simulink model "PP_simulink_Sily"  (R2024b)
settings: Solver=ode1  StartTime=0.0  StopTime=1  FixedStep=0.005  RelTol=1e-3
values from neighbouring files (symbols this model uses):
  init_int_dref = -Ki\((Uinit-Us)+Kp*(Xinit_ss-Xs))    [PP_matlab_client_Sily.m]
  Ki = K_ex_other_angles(:, 17:20)    [PP_koeficienty.m]
  Kp = K_ex_other_angles(:, 1:16)    [PP_koeficienty.m]
  L_obs = place(Ac', Cc', poles_obs)'    [PP_koeficienty.m]
undefined symbols (not defined in the file or in its folder): b_moment, d, g, Ip, Ixx, Iyy, Izz, k_thrust, l, M, m, Us, Xinit_ss, Xs
libraries: simulink_extras x6
settings Model: Creator=yaozhong.zhang  LastModifiedBy=Admin
settings DebuggingCC: UnconnectedInputMsg=warning  UnconnectedOutputMsg=warning  UnconnectedLineMsg=warning
settings ModelReferenceCC: EnableRefExpFcnMdlSchedulingChecks=on
settings RTWCC: GPUComputeCapability=3.5

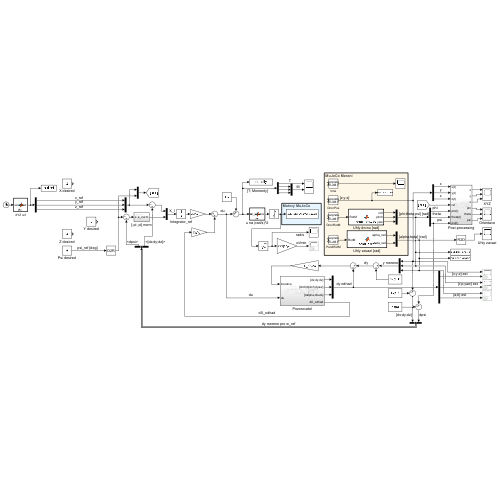
[thumbnail: Simulink's stored preview of the top-level diagram]
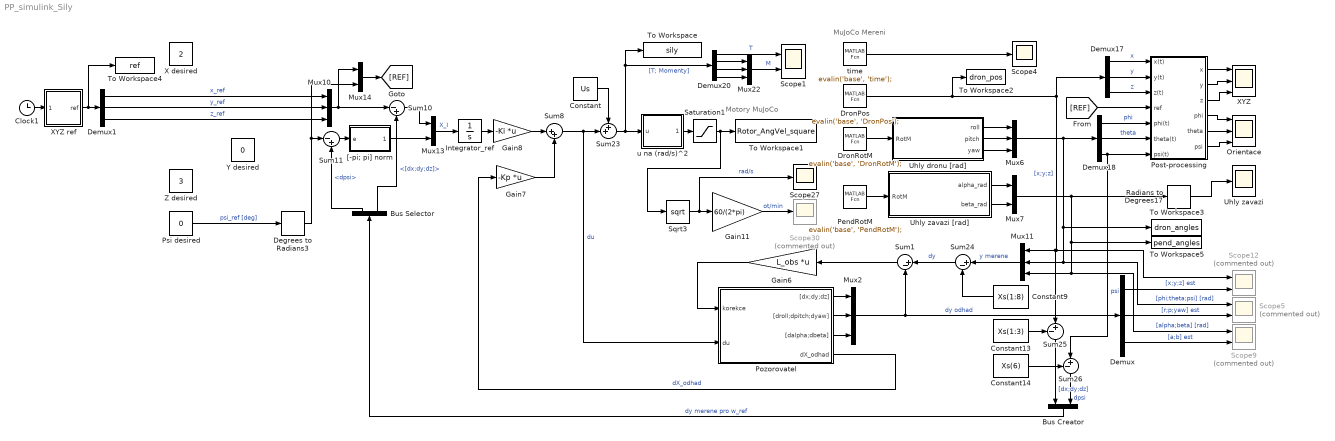
== system PP_simulink_Sily ==
  note: Motory MuJoCo
  note: MuJoCo Mereni
  Bus Creator : BusCreator  Inputs=2
  Bus Selector : BusSelector  OutputSignals=dpsi,[dx;dy;dz]
  Clock1 : Clock
  Constant : Constant  Value=Us
  Constant13 : Constant  Value=Xs(1:3)
  Constant14 : Constant  Value=Xs(6)
  Constant9 : Constant  Value=Xs(1:8)
  Degrees to Radians3 : simulink_extras/Transformations/Degrees to Radians
  Demux{,1,17..18} (4 alike) : Demux  Outputs=3
  Demux20 : Demux
  DronPos : MATLABFcn  MATLABFcn=evalin('base', 'DronPos');  OutputDimensions=[3,1]  Output1D=off
  DronRotM : MATLABFcn  MATLABFcn=evalin('base', 'DronRotM');  OutputDimensions=[3,3]  Output1D=off
  Gain11 : Gain  Gain=60/(2*pi)
  Gain6 : Gain  Gain=L_obs  Multiplication=Matrix(K*u)
  Gain7 : Gain  Gain=-Kp  Multiplication=Matrix(K*u)
  Gain8 : Gain  Gain=-Ki  Multiplication=Matrix(K*u)
  Integrator_ref : Integrator  InitialCondition=init_int_dref
  Mux{2,6,10..11,22} (5 alike) : Mux  Inputs=3
  Mux13 : Mux  Inputs=2
  Mux14 : Mux  Inputs=2
  Mux7 : Mux  Inputs=2
  Orientace : Scope  NumInputPorts=3
  PendRotM : MATLABFcn  MATLABFcn=evalin('base', 'PendRotM');  OutputDimensions=[3,3]  Output1D=off
  Post-processing : Subsystem
  Pozorovatel : Subsystem
  Psi desired : Constant  Value=0
  Radians to Degrees17 : simulink_extras/Transformations/Radians to Degrees
  Saturation1 : Saturate  UpperLimit=1976^2  LowerLimit=0
  Scope1 : Scope  NumInputPorts=2
  Scope12 : Scope  Commented=on  NumInputPorts=2
  Scope27 : Scope
  Scope30 : Scope  Commented=on
  Scope4 : Scope
  Scope5 : Scope  Commented=on  NumInputPorts=2
  Scope9 : Scope  Commented=on  NumInputPorts=2
  Sqrt3 : Sqrt
  Sum1 : Sum  Inputs=|+-
  Sum10 : Sum  Inputs=|-+
  Sum11 : Sum  Inputs=|-+
  Sum23 : Sum  Inputs=++|
  Sum24 : Sum  Inputs=|+-
  Sum25 : Sum  Inputs=-+|
  Sum26 : Sum  Inputs=-+|
  Sum8 : Sum  Inputs=|++
  To Workspace : ToWorkspace  VariableName=sily  SaveFormat=Timeseries  SampleTime=-1
  To Workspace1 : ToWorkspace  VariableName=Rotor_AngVel_square  SampleTime=-1
  To Workspace2 : ToWorkspace  VariableName=dron_pos  SaveFormat=Timeseries  SampleTime=-1
  To Workspace3 : ToWorkspace  VariableName=dron_angles  SaveFormat=Timeseries  SampleTime=-1
  To Workspace4 : ToWorkspace  VariableName=ref  SaveFormat=Timeseries  SampleTime=-1
  To Workspace5 : ToWorkspace  VariableName=pend_angles  SaveFormat=Timeseries  SampleTime=-1
  Uhly dronu [rad] : MATLAB Function  TreatAsAtomicUnit=on
  Uhly zavazi : Scope
  Uhly zavazi [rad] : MATLAB Function  TreatAsAtomicUnit=on
  X desired : Constant  Value=2
  XYZ : Scope  NumInputPorts=3
  XYZ ref : MATLAB Function  TreatAsAtomicUnit=on
  Y desired : Constant  Value=0
  Z desired : Constant  Value=3
  "[-pi; pi] norm" : Subsystem
  time : MATLABFcn  MATLABFcn=evalin('base', 'time');  Output1D=off
  u na (rad/s)^2 : MATLAB Function  TreatAsAtomicUnit=on
  wires:
  Demux/1 -> Scope12/2  "[x;y;z] est"
  Demux/2 -> Scope5/2  "[r;p;yaw] est"
  Demux/3 -> Scope9/2  "[a;b] est"
  Mux6/1 -> Mux11/2, Scope5/1, To Workspace3/1, Demux18/1  "[phi;theta;psi] [rad]"
  Gain7/1 -> Sum8/2
  Post-processing/1(x) -> XYZ/1
  Integrator_ref/1 -> Gain8/1
  Post-processing/5(theta) -> Orientace/2
  Degrees to Radians3/1 -> Mux14/2, Sum11/1
  Post-processing/4(phi) -> Orientace/1
  [REF] -> Post-processing/4(ref)
  Mux13/1 -> Integrator_ref/1  "X_I"
  Demux17/1 -> Post-processing/1(x(t))  "x"
  Radians to Degrees17/1 -> Uhly zavazi/1
  Mux22/1 -> Scope1/2  "M"
  Gain11/1 -> Scope30/1  "ot/min"
  Post-processing/6(psi) -> Orientace/3
  Demux18/1 -> Post-processing/5(phi(t))  "phi"
  Sqrt3/1 -> Scope27/1, Gain11/1  "rad/s"
  Pozorovatel/4(dX_odhad) -> Gain7/1  "dX_odhad"
  Demux18/3 -> Post-processing/7(psi(t)), Sum26/2  "psi"
  Demux1/3 -> Mux10/3  "z_ref"
  Post-processing/3(z) -> XYZ/3
  "[-pi; pi] norm"/1(e_norm) -> Mux13/2
  Sum10/1 -> Mux13/1
  Demux18/2 -> Post-processing/6(theta(t))  "theta"
  Psi desired/1 -> Degrees to Radians3/1  "psi_ref [deg]"
  Demux20/4 -> Mux22/3
  Demux20/1 -> Scope1/1  "T"
  Post-processing/2(y) -> XYZ/2
  Sum23/1 -> To Workspace/1, Demux20/1, u na (rad/s)^2/1(u)  "[T; Momenty]"
  Bus Creator/1 -> Bus Selector/1  "dy merene pro w_ref"
  Gain8/1 -> Sum8/1
  Demux1/1 -> Mux10/1  "x_ref"
  Sum11/1 -> "[-pi; pi] norm"/1(e)
  Demux20/3 -> Mux22/2
  Demux17/3 -> Post-processing/3(z(t))  "z"
  Mux10/1 -> Mux14/1, Sum10/1
  DronPos/1 -> To Workspace2/1, Demux17/1, Mux11/1, Sum25/2, Scope12/1  "[x;y;z]"
  Demux1/2 -> Mux10/2  "y_ref"
  Demux20/2 -> Mux22/1
  Demux17/2 -> Post-processing/2(y(t))  "y"
  u na (rad/s)^2/1(wi_square) -> Saturation1/1
  Saturation1/1 -> Sqrt3/1, To Workspace1/1
  Uhly zavazi [rad]/1(alpha_rad) -> Mux7/1
  time/1 -> Scope4/1
  Uhly zavazi [rad]/2(beta_rad) -> Mux7/2
  Mux7/1 -> Radians to Degrees17/1, Mux11/3, Scope9/1, To Workspace5/1  "[alpha;beta] [rad]"
  DronRotM/1 -> Uhly dronu [rad]/1(RotM)
  Uhly dronu [rad]/1(roll) -> Mux6/1
  Uhly dronu [rad]/3(yaw) -> Mux6/3
  Uhly dronu [rad]/2(pitch) -> Mux6/2
  PendRotM/1 -> Uhly zavazi [rad]/1(RotM)
  Mux14/1 -> [REF]
  Sum25/1 -> Bus Creator/1  "[dx;dy;dz]"
  Constant13/1 -> Sum25/1
  Constant14/1 -> Sum26/1
  Sum26/1 -> Bus Creator/2  "dpsi"
  Bus Selector/1 -> Sum11/2  "<dpsi>"
  Bus Selector/2 -> Sum10/2  "<[dx;dy;dz]>"
  Constant/1 -> Sum23/1
  Sum8/1 -> Pozorovatel/2(du), Sum23/2  "du"
  Sum24/1 -> Sum1/1  "dy"
  Mux2/1 -> Sum1/2, Demux/1  "dy odhad"
  Gain6/1 -> Pozorovatel/1(korekce)
  Mux11/1 -> Sum24/1  "y merene"
  Constant9/1 -> Sum24/2
  Sum1/1 -> Gain6/1
  Pozorovatel/1("[dx;dy;dz]") -> Mux2/1
  Pozorovatel/2("[droll;dpitch;dyaw]") -> Mux2/2
  Pozorovatel/3("[dalpha;dbeta]") -> Mux2/3
  Clock1/1 -> XYZ ref/1(simtime)
  XYZ ref/1(ref) -> To Workspace4/1, Demux1/1

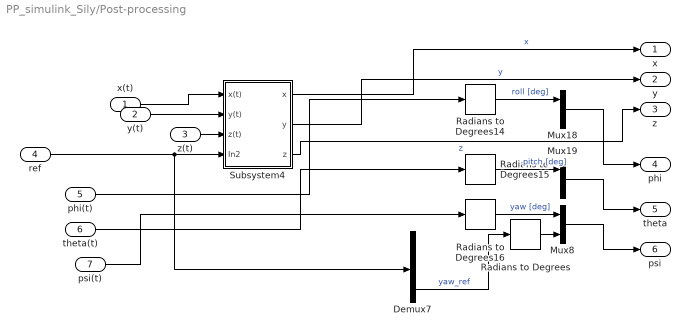
== system PP_simulink_Sily/Post-processing ==
  x(t) : Inport
  y(t) : Inport  Port=2
  z(t) : Inport  Port=3
  ref : Inport  Port=4
  phi(t) : Inport  Port=5
  theta(t) : Inport  Port=6
  psi(t) : Inport  Port=7
  Demux7 : Demux
  Mux18 : Mux  Inputs=2
  Mux19 : Mux  Inputs=2
  Mux8 : Mux  Inputs=2
  Radians to Degrees{,14..16} (4 alike) : simulink_extras/Transformations/Radians to Degrees
  Subsystem4 : Subsystem
  x : Outport
  y : Outport  Port=2
  z : Outport  Port=3
  phi : Outport  Port=4
  theta : Outport  Port=5
  psi : Outport  Port=6
  wires:
  Radians to Degrees16/1 -> Mux8/1  "yaw [deg]"
  ref/1 -> Subsystem4/4(In2), Demux7/1
  Demux7/4 -> Radians to Degrees/1  "yaw_ref"
  theta(t)/1 -> Radians to Degrees15/1
  Mux18/1 -> phi/1
  Subsystem4/3(z) -> z/1  "z"
  Radians to Degrees14/1 -> Mux18/1  "roll [deg]"
  Radians to Degrees15/1 -> Mux19/1  "pitch [deg]"
  Subsystem4/2(y) -> y/1  "y"
  x(t)/1 -> Subsystem4/1(x(t))
  y(t)/1 -> Subsystem4/2(y(t))
  psi(t)/1 -> Radians to Degrees16/1
  phi(t)/1 -> Radians to Degrees14/1
  Subsystem4/1(x) -> x/1  "x"
  Mux8/1 -> psi/1
  z(t)/1 -> Subsystem4/3(z(t))
  Mux19/1 -> theta/1
  Radians to Degrees/1 -> Mux8/2

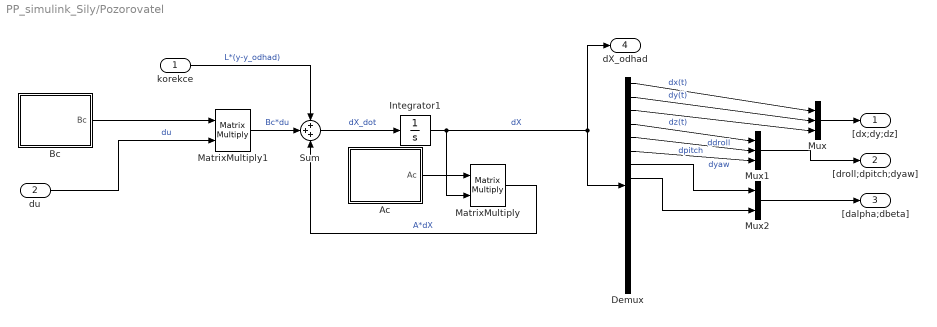
== system PP_simulink_Sily/Pozorovatel ==
  korekce : Inport
  du : Inport  Port=2
  Ac : MATLAB Function  TreatAsAtomicUnit=on
  Bc : MATLAB Function  TreatAsAtomicUnit=on
  Demux : Demux  Outputs=16
  Integrator1 : Integrator  InitialCondition=Xinit_ss - Xs
  MatrixMultiply : Product  Multiplication=Matrix(*)
  MatrixMultiply1 : Product  Multiplication=Matrix(*)
  Mux : Mux  Inputs=3
  Mux1 : Mux  Inputs=3
  Mux2 : Mux  Inputs=2
  Sum : Sum  Inputs=+++
  "[dx;dy;dz]" : Outport
  "[droll;dpitch;dyaw]" : Outport  Port=2
  "[dalpha;dbeta]" : Outport  Port=3
  dX_odhad : Outport  Port=4
  wires:
  du/1 -> MatrixMultiply1/2  "du"
  Ac/1(Ac) -> MatrixMultiply/1
  Integrator1/1 -> Demux/1, dX_odhad/1, MatrixMultiply/2  "dX"
  Demux/1 -> Mux/1  "dx(t)"
  Demux/2 -> Mux/2  "dy(t)"
  Demux/3 -> Mux/3  "dz(t)"
  Mux/1 -> "[dx;dy;dz]"/1
  Demux/4 -> Mux1/1  "ddroll"
  Demux/5 -> Mux1/2  "dpitch"
  Demux/6 -> Mux1/3  "dyaw"
  Mux1/1 -> "[droll;dpitch;dyaw]"/1
  Sum/1 -> Integrator1/1  "dX_dot"
  MatrixMultiply1/1 -> Sum/2  "Bc*du"
  MatrixMultiply/1 -> Sum/3  "A*dX"
  Bc/1(Bc) -> MatrixMultiply1/1
  Mux2/1 -> "[dalpha;dbeta]"/1
  Demux/7 -> Mux2/1
  Demux/8 -> Mux2/2
  korekce/1 -> Sum/1  "L*(y-y_odhad)"

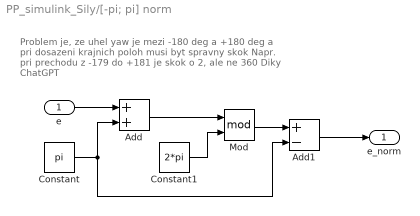
== system PP_simulink_Sily/[-pi; pi] norm ==
  note: Problem je, ze uhel yaw je mezi -180 deg a +180 deg
      | a pri dosazeni krajnich poloh musi byt spravny skok
      | Napr. pri prechodu z -179 do +181 je skok o 2, ale ne 360
      | Diky ChatGPT
  e : Inport
  Add : Sum
  Add1 : Sum  Inputs=+-
  Constant : Constant  Value=pi
  Constant1 : Constant  Value=2*pi
  Mod : Math  Operator=mod
  e_norm : Outport
  wires:
  e/1 -> Add/1
  Add/1 -> Mod/1
  Constant/1 -> Add1/2, Add/2
  Constant1/1 -> Mod/2
  Mod/1 -> Add1/1
  Add1/1 -> e_norm/1

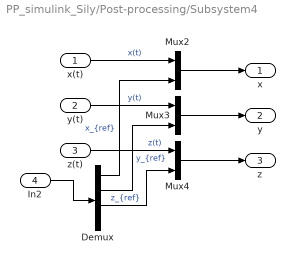
== system PP_simulink_Sily/Post-processing/Subsystem4 ==
  x(t) : Inport
  y(t) : Inport  Port=2
  z(t) : Inport  Port=3
  In2 : Inport  Port=4
  Demux : Demux
  Mux2 : Mux  Inputs=2
  Mux3 : Mux  Inputs=2
  Mux4 : Mux  Inputs=2
  x : Outport
  y : Outport  Port=2
  z : Outport  Port=3
  wires:
  Demux/2 -> Mux3/2  "y_{ref}"
  Mux4/1 -> z/1
  y(t)/1 -> Mux3/1  "y(t)"
  Mux3/1 -> y/1
  Demux/1 -> Mux2/2  "x_{ref}"
  Demux/3 -> Mux4/2  "z_{ref}"
  Mux2/1 -> x/1
  In2/1 -> Demux/1
  x(t)/1 -> Mux2/1  "x(t)"
  z(t)/1 -> Mux4/1  "z(t)"

== matlab function PP_simulink_Sily/Uhly dronu [rad] ==
  data: RotM input; roll output; pitch output; yaw output
function [roll, pitch, yaw] = quad_attitude(RotM)
% matice rotace koptery z Python, vuci svetu!!!
% rotm2eul prevadi na Eulerove uhly
radians = rotm2eul(RotM, 'ZYX'); % pouzivam poradi ZYX

% roll = kolem x, pitch = kolem y, yaw = kolem z
yaw = radians(1);
pitch = radians(2);
roll = radians(3);
end

== matlab function PP_simulink_Sily/Pozorovatel/Ac ==
  data: g parameter; M parameter; Ac output; m parameter; Ip parameter; d parameter
function Ac = fcn(g, M, m, Ip, d)
% Matice Ac linearizovana kvadrokoptera+zavazi

Ac = [
0, 0, 0,                 0,                  0, 0,                  0,                  0, 1, 0, 0, 0, 0, 0, 0, 0;
0, 0, 0,                 0,                  0, 0,                  0,                  0, 0, 1, 0, 0, 0, 0, 0, 0;
0, 0, 0,                 0,                  0, 0,                  0,                  0, 0, 0, 1, 0, 0, 0, 0, 0;
0, 0, 0,                 0,                  0, 0,                  0,                  0, 0, 0, 0, 1, 0, 0, 0, 0;
0, 0, 0,                 0,                  0, 0,                  0,                  0, 0, 0, 0, 0, 1, 0, 0, 0;
0, 0, 0,                 0,                  0, 0,                  0,                  0, 0, 0, 0, 0, 0, 1, 0, 0;
0, 0, 0,                 0,                  0, 0,                  0,                  0, 0, 0, 0, 0, 0, 0, 1, 0;
0, 0, 0,                 0,                  0, 0,                  0,                  0, 0, 0, 0, 0, 0, 0, 0, 1;
0, 0, 0,                 0,      (g*(M + m))/M, 0,            (g*m)/M,                  0, 0, 0, 0, 0, 0, 0, 0, 0;
0, 0, 0,    -(g*(M + m))/M,                  0, 0,                  0,            (g*m)/M, 0, 0, 0, 0, 0, 0, 0, 0;
0, 0, 0,                 0,                  0, 0,                  0,                  0, 0, 0, 0, 0, 0, 0, 0, 0;
0, 0, 0,                 0,                  0, 0,                  0,                  0, 0, 0, 0, 0, 0, 0, 0, 0;
0, 0, 0,                 0,                  0, 0,                  0,                  0, 0, 0, 0, 0, 0, 0, 0, 0;
0, 0, 0,                 0,                  0, 0,                  0,                  0, 0, 0, 0, 0, 0, 0, 0, 0;
0, 0, 0,                 0, -(g*(M + m))/(M*d), 0, -(g*(M + m))/(M*d),                  0, 0, 0, 0, 0, 0, 0, 0, 0;
0, 0, 0, (g*(M + m))/(M*d),                  0, 0,                  0, -(g*(M + m))/(M*d), 0, 0, 0, 0, 0, 0, 0, 0];

== matlab function PP_simulink_Sily/Pozorovatel/Bc ==
  data: M parameter; Bc output; Ixx parameter; Iyy parameter; Izz parameter; m parameter
function Bc = fcn(M, Ixx, Iyy, Izz, m)
% Matice Ac linearizovana

Bc = [
        0,     0,     0,     0;
        0,     0,     0,     0;
        0,     0,     0,     0;
        0,     0,     0,     0;
        0,     0,     0,     0;
        0,     0,     0,     0;
        0,     0,     0,     0;
        0,     0,     0,     0;
        0,     0,     0,     0;
        0,     0,     0,     0;
1/(M + m),     0,     0,     0;
        0, 1/Ixx,     0,     0;
        0,     0, 1/Iyy,     0;
        0,     0,     0, 1/Izz;
        0,     0,     0,     0;
        0,     0,     0,     0];

== matlab function PP_simulink_Sily/XYZ ref ==
  data: ref output; simtime input
function ref = fcn(simtime)
% pouze poloha, yaw_ref=0
if simtime < 1
    ref = [0;0;2];
elseif simtime < 6
    ref = [3;3;2];
elseif simtime < 10
    ref = [3;3;6];
elseif simtime < 15
    ref = [3;0;6];
elseif simtime < 22
    ref = [3;-3;8];
elseif simtime < 30
    ref = [-3;0;6];
elseif simtime < 35
    ref = [-3;3;6];
elseif simtime < 38
    ref = [-3;3;3];
elseif simtime < 40
    ref = [0;3;2];
elseif simtime < 45 % -> simtime 50s
    ref = [0;0;2];
else
    ref = [0;0;2]; % pokud co, tak pocatecni poloha
end

== matlab function PP_simulink_Sily/Uhly zavazi [rad] ==
  data: RotM input; alpha_rad output; beta_rad output
function [alpha_rad, beta_rad] = pend_orient(RotM)
% Расчет углов альфа и бета маятника

% Вектор маятника
rope_vector = RotM * [0; 0; -1];

% Расчет угла альфа
rope_vector_xz = rope_vector([1, 3]); % Компоненты x и z
z_axis = [0; -1];
cos_alpha = dot(rope_vector_xz, z_axis) / (norm(rope_vector_xz) * norm(z_axis));
cos_alpha = max(-1, min(1, cos_alpha)); % Ограничиваем в диапазоне [-1, 1]
alpha = acos(cos_alpha);
if rope_vector(1) < 0
    alpha = -alpha;
end

% Расчет угла бета
rope_vector_xz_3 = [rope_vector(1); 0; rope_vector(3)];
cos_beta = dot(rope_vector, rope_vector_xz_3) / (norm(rope_vector) * norm(rope_vector_xz_3));
cos_beta = max(-1, min(1, cos_beta)); % Ограничиваем в диапазоне [-1, 1]
beta = acos(cos_beta);
if rope_vector(2) < 0
    beta = -beta;
end

% Округляем до 5 знаков после запятой
% alpha_rad = round(alpha, 5); %[rad]
% beta_rad = round(beta, 5); %[rad]
alpha_rad = alpha;
beta_rad = beta;

== matlab function PP_simulink_Sily/u na (rad//s)^2 ==
  data: u input; wi_square output; b_moment parameter; k_thrust parameter; l parameter
function wi_square = fcn(u, b_moment, k_thrust, l)

T = u(1);
Tau_phi = u(2);
Tau_theta = u(3);
Tau_psi = u(4);

w1 = ( (Tau_phi*b_moment - Tau_theta*b_moment + l*T*b_moment + l*Tau_psi*k_thrust)/(4*l*b_moment*k_thrust));
w2 = ( (-Tau_theta*b_moment - Tau_phi*b_moment + l*T*b_moment - l*Tau_psi*k_thrust)/(4*l*b_moment*k_thrust));
w3 = ( (Tau_theta*b_moment - Tau_phi*b_moment + l*T*b_moment + l*Tau_psi*k_thrust)/(4*l*b_moment*k_thrust));
w4 = ( (Tau_phi*b_moment + Tau_theta*b_moment + l*T*b_moment - l*Tau_psi*k_thrust)/(4*l*b_moment*k_thrust));

wi_square = [w1;w2;w3;w4];
